simulink model "LookupTableND_3D_2"  (R2017b)
settings: Solver=FixedStepDiscrete  StartTime=0.0  StopTime=10.0  FixedStep=0.200000  RelTol=1e-3  EnableMultiTasking=on
model workspace (MAT data in the model file):
  T = reshape([0.652225769628 0.345744878699 -0.344685690214 0.0307859462286 -0.133347855387 -0.626037347851 1.11143973329 1.2021662592 0.0723818568121 -1.0267475714 -1.17297048771 0.25100421714 -0.264622209197 -0.81319077394 0.132016782961 -1.18465169495 0.340420554323 -1.59209341809 -2.45376333568 -0.208120578004 -0.981929884247 1.53111911749 1.37266970097 -0.612117906862 -0.966737022546 -0.216395399401 -0.316082461732], [3 3 3])
settings Model: Creator=hbourbou  LastModifiedBy=hbourbou
settings DataIOCC: LimitDataPoints=on  SaveFormat=StructureWithTime
settings OptimizationCC: LifeSpan=inf
settings DebuggingCC: SFUnexpectedBacktrackingDiag=warning  SFNoUnconditionalDefaultTransitionDiag=warning  SFExecutionAtInitializationDiag=none
settings HardwareCC: ProdBitPerSizeT=32  ProdBitPerPtrDiffT=32  ProdWordSize=32  ProdHWDeviceType=Specified
settings ModelReferenceCC: PropagateSignalLabelsOutOfModel=off
settings CodeAppCC: StateflowObjectComments=on
settings GRTTargetCC: TargetLangStandard=C89/C90 (ANSI)
settings ConfigComp: CovMetricSettings=dw  CovHtmlReporting=on  CovSaveCumulativeToWorkspaceVar=on  CovSaveSingleToWorkspaceVar=on  CovExternalEMLEnable=off

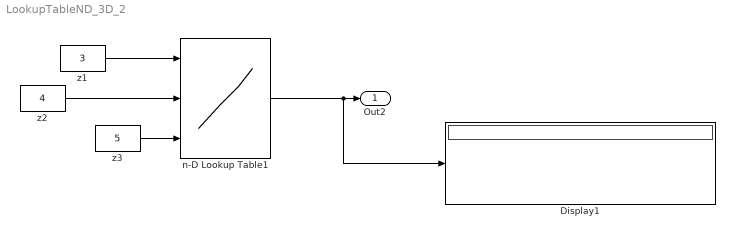
== system LookupTableND_3D_2 ==
  Display1 : Display
  n-D Lookup Table1 : Lookup_n-D  NumberOfTableDimensions=3  BreakpointsForDimension1=[1 2 4]  BreakpointsForDimension2=[1 3 4]  BreakpointsForDimension3=[1 2 3 ]  Table=T  InternalRulePriority=Speed  RndMeth=Simplest  InputSameDT=on
  z1 : Constant  Value=3
  z2 : Constant  Value=4
  z3 : Constant  Value=5
  Out2 : Outport
  wires:
  z1/1 -> n-D Lookup Table1/1
  n-D Lookup Table1/1 -> Out2/1, Display1/1
  z2/1 -> n-D Lookup Table1/2
  z3/1 -> n-D Lookup Table1/3
